simulink model "AME556_Project_Task5"  (R2024b)
settings: Solver=daessc  StartTime=0.0  StopTime=5  FixedStep=0.0005  MaxStep=1e-3  RelTol=1e-2
InitFcn:
  | global params;
  | 
  | % Mass and geometry
  | params.m = 0.25;
  | params.l = 0.22;
  | params.mb = 8;
  | params.a = 0.25;
  | params.b = 0.15;
  | params.g = [0; 9.81; 0];
  | 
  | % Moment of inerita
  | Il_zz = params.m * params.l^2 / 12;
  | Ib_xx = params.mb * params.a^2 / 12;
  | Ib_yy = params.mb * params.b^2 / 12;
  | Ib_zz = params.mb * (params.a^2 + params.b^2) / 12;
  | params.Ib = diag([Ib_xx Ib_yy Ib_zz]);
  | 
  | % Spatial contact force parameters
  | Kp_g = 1e5;
  | Kd_g = 1e3;
  | 
  | % Ground contact positions
  | params.P1 = [0.0197; 0.0022; 0];
  | params.P2 = [0.1838; 0.0041; 0];
  | 
  | % State variables
  | q0 = [0.1; 0.45; 0; -pi/3; pi/2; -pi/6; pi/2]; % Initial states (before landing)
  | params.p_d = [0; 0.5; 0]; % Desired positions (after standing): [x_d; y_d; z_d];
  | params.theta_d = 0; % Desired angle
values from neighbouring files (symbols this model uses):
  dt = 0.04    [AME556_Project_Task5_Setup.m]
  l = 0.5    [AME556_Project_Task5_Setup.m]
  N = 10    [AME556_Project_Task5_Setup.m]
undefined symbols (not defined in the file or in its folder): P1_world0, P2_world0, X, Y, Z
libraries: sm_lib x33, nesl_utility x27
(part 2 of 2)

== matlab function AME556_Project_Task5/MATLAB Function ==
  data: tau_unsaturated input; tau_saturated output; saturateSwitch input
function tau_saturated = tau_saturation(tau_unsaturated, saturateSwitch)
    if saturateSwitch == 1
        tau_limits = [30, 60, 30, 60];
    
        tau_saturated = tau_unsaturated;
    
        for i = 1:length(tau_unsaturated)
            if tau_unsaturated(i) > tau_limits(i)
                tau_saturated(i) = tau_limits(i);
                warning('Tau %d (%.2f) is saturated to %d', i, tau_unsaturated(i), tau_limits(i));
            elseif tau_unsaturated(i) < -tau_limits(i)
                tau_saturated(i) = -tau_limits(i);
                warning('Tau %d (%.2f) is saturated to -%d', i, tau_unsaturated(i), tau_limits(i));
            end
        end
    else
        tau_saturated = tau_unsaturated;
    end
end

== matlab function AME556_Project_Task5/Controller/Condensed MPC Controller ==
  data: p input; theta input; dp input; dtheta input; qs input; tau output; P1 input; P2 input; dP1 input; dP2 input; N input; dt input; t input
%% Function: Low Level Control

function tau = lowLevelControl(p, theta, dp, dtheta, qs, P1, P2, dP1, dP2, N, dt, t)

% 步态的行为应该有：walk run stairs jump_onto_obstacle jump_onto_floor jump_over_pit

if p(1) < 1.8 
    % walk (0,1.8)
    gaitType = "walk";
elseif p(1) < 2.8
    % jump_onto_obstacle (1.8,2.8)
    gaitType = "jump";
elseif p(1) < 4.8
    % jump_onto_floor (2.8,3.8)
elseif p(1) < 5.2
    % jump_over_pit (3.8,4.4)
else
    % walk (4.4,~)
end

con = gaitSchedule(N, dt, t, gaitType);
F = condensed_mpc_controller(p, theta, dp, dtheta, P1, P2, N, dt, t, con, gaitType);
J = jacobianFcn(theta, qs);

tau = zeros(4, 1);
if con(1, 1) && con(2, 1)
    tau = -J' * F;
elseif con(1, 1) && ~con(2, 1)
    F_swing = swingLegControl(p, dp, P2, dP2, N, dt, t, gaitType);
    F_new = [F(1: 2); -F_swing];
    tau = -J' * F_new;
elseif con(2, 1) && ~con(1, 1)
    F_swing = swingLegControl(p, dp, P1, dP1, N, dt, t, gaitType);
    F_new = [-F_swing; F(3: 4)];
    tau = -J' * F_new;    
else
    % 为了飞的修改：俩腿都swing
    F_swing1 = swingLegControl(p, dp, P1, dP1, N, dt, t, gaitType);
    F_swing2 = swingLegControl(p, dp, P2, dP2, N, dt, t, gaitType);
    F_new = [-F_swing1; -F_swing2];
    tau = -J' * F_new;
    % 飞行修改结束
end

end

%% Function: Condensed MPC Controller

function F = condensed_mpc_controller(p, theta, dp, dtheta, P1, P2, N, dt, t, con, gaitType)

    % 为了飞的修改：~any(con(:, 1)) 任何一条腿都不为1（也就是都是0）的话，直接F=0
    if ~any(con(:, 1))
        F = zeros(4, 1); 
        return;
    end
    % 为了飞的修改结束

% Parameters
mt = 8;
a = 0.25;
b = 0.15;
g = [0; 9.81; 0];
Ib_zz = mt * (a^2 + b^2) / 12;

numStates = 7;
numCtrls = 4;
Q = diag([200 200 800 30 10 10 0]);
R = 0.0001*eye(numCtrls);

% q = [x; y; z; R1; dx; dy; dz; wbx; wby; wbz];
% X = [x; y; theta; dx; dy; dtheta; g];
X = zeros(numStates, 1);
X(1: 2) = p;
X(3) = theta;
X(4: 5) = dp;
X(6) = dtheta;
X(7) = g(2);

% Desired states
if gaitType == "walk"
    if t < 1
        X_d = [p_d(1); 0.45; 0; t; 0; 0; g(2)]; % Lower ground walking (acceleration)
    else
        X_d = [p_d(1); 0.45; 0; 1; 0; 0; g(2)]; % Lower ground walking (constant speed)
    end
elseif gaitType == "jump"
    X_d = [p_d(1); 0.4 + 0.45; 0; 1; 0.5; 0; g(2)]; % Going upstairs
end

% Reference Trajectory
X_ref = getReferenceTrajectory(dt, N, p, theta, dp, dtheta, X_d);
y = reshape(X_ref, [numStates*N 1]);

r1 = P1 - p;
r2 = P2 - p;

% Linearized system (A, B)
A = [zeros(3)   eye(3)    zeros(3,1);
     zeros(3, numStates-1) [0; -1; 0];
     zeros(1, numStates)];

B = [zeros(3, numCtrls);
     eye(2)/mt eye(2)/mt;
     -r1(2)/Ib_zz r1(1)/Ib_zz -r2(2)/Ib_zz r2(1)/Ib_zz;
     zeros(1, numCtrls)];

% Discrete-time system matrices (Ak, Bk)
Ak = A * dt + eye(size(A, 1));
Bk = B * dt;

% Aqp
Aqp = [];
for i = 1: N
    Aqp = [Aqp; mpower(Ak, i)];
end

% bqp
Bqp = repmat(zeros(size(Bk)), N, N);
for i = 0: N-1
    element = mpower(Ak, i) * Bk;
    Bqp = Bqp + kron(diag(ones(1, N - i), -i), element);
end

% Condensation
L = kron(eye(N), Q);
K = kron(eye(N), R);

% Optimization weights (H, f)
H = 2*(Bqp'*L*Bqp + K);
f = 2*Bqp'*L*(Aqp*X - y);

% Inequality constraints (A_ineq, b_ineq)
Aineq_mu = kron(eye(2), [1 -0.7; -1 -0.7]);
Aineq_mu_N = kron(eye(N), Aineq_mu);
Aineq_F = kron(eye(2), [0 1; 0 -1]);
Aineq_F_N = kron(eye(N), Aineq_F);
Aineq = [Aineq_mu_N; Aineq_F_N];

bineq_mu = repmat([0; 0; 0; 0], N, 1);
bineq_f = [];
for i = 1: N
    bineq_f = [bineq_f; [250; -10]*con(1, i); [250; -10]*con(2, i)];
end
bineq = [bineq_mu; bineq_f];

% Initial guess
u0 = zeros(length(f), 1);

% Quadratic programming
options = optimoptions('quadprog', 'Algorithm', 'active-set', 'Display', 'off');
u_mpc = quadprog(H, f, Aineq, bineq, [], [], [], [], u0, options);

% Force inputs
F = u_mpc(1: numCtrls);

end

%% Function: Get Reference Geometry

function X_ref = getReferenceTrajectory(dt, N, p, theta, dp, dtheta, X_d)

X = [p; theta; dp; dtheta; 9.81];
X_ref = repmat(X, 1, N);

for i = 1: 3
    for k = 2: N
        if X_d(i + 3) ~= 0
            X_ref(i, k) = X(i) + X_d(i+3)*((k-1)*dt);
        else
            X_ref(i, k) = X_d(i);
        end
    end
end

end

%% Function: Swing Leg Control

function F_swing = swingLegControl(p, dp, P_swing, dP_swing, P_support, N, dt, t)

Kp = diag([200 300]);
Kd = eye(2)*5;

del_t = N*dt/2; % Time duration of swing phase
ts = rem(t, N*dt/2);

if gaitType == "walk"
    swingHeight = 0.1;
    Px_d = p(1) + (1/2)*del_t*dp(1);
    Py_d = swingHeight * sin(pi*ts/del_t); % Flat ground walking
    disp('walk')

elseif gaitType == "jump"
    swingHeight = 0.4;
    Px_d = p(1) + (1/2)*del_t*dp(1);
    Py_d = P_support(2) + (1/2)*del_t*dp(2) + 2*(sin(pi*ts/del_t))^(1/3)*swingHeight; % Going upstairs
    disp('climb')
    
end

F_swing = Kp*([Px_d; Py_d] - P_swing) + Kd*(0 - dP_swing);

end

%% Function: Jacobian Function
% Convert contact forces to joint torques

function J = jacobianFcn(theta, qs)

l = 0.22;

q1 = qs(1); q2 = qs(2); q3 = qs(3); q4 = qs(4);

J = [l*cos(q1 + q2 + theta) + l*cos(q1 + theta), l*cos(q1 + q2 + theta),                                          0,                      0;
     l*sin(q1 + q2 + theta) + l*sin(q1 + theta), l*sin(q1 + q2 + theta),                                          0,                      0;
                                              0,                      0, l*cos(q3 + q4 + theta) + l*cos(q3 + theta), l*cos(q3 + q4 + theta);
                                              0,                      0, l*sin(q3 + q4 + theta) + l*sin(q3 + theta), l*sin(q3 + q4 + theta)];

end

%% Function: Gait Schedule
% Generate gait schedule based on walking phase

function sigma = gaitSchedule(N, dt, t, gaitType)

    if gaitType == "walk"
        phase = floor(t/dt);
        k = rem(phase, N);
        
        sigma_l0 = [ones(1, N/2) zeros(1, N/2)];
        sigma_r0 = [zeros(1, N/2) ones(1, N/2)];
        
        if k ~= 0
            sigma_l = [sigma_l0(k+1: N) sigma_l0(1: k)];
            sigma_r = [sigma_r0(k+1: N) sigma_r0(1: k)];
        else
            sigma_l = sigma_l0;
            sigma_r = sigma_r0;
        end
        
        sigma = [sigma_l; sigma_r];

    elseif gaitType == "jump"
        phase = floor(t/dt);
        k = rem(phase, N);
        
        sigma_l0 = [1 1 1 1 1 0 0 0 0 0];
        sigma_r0 = [1 1 1 1 1 0 0 0 0 0];
        
        if k ~= 0
            sigma_l = [sigma_l0(k+1: N) sigma_l0(1: k)];
            sigma_r = [sigma_r0(k+1: N) sigma_r0(1: k)];
        else
            sigma_l = sigma_l0;
            sigma_r = sigma_r0;
        end
        
        sigma = [sigma_l; sigma_r];       
    
    end
end

== matlab function AME556_Project_Task5/MATLAB Function1 ==
  data: dq input
function physicalConstrains(dq) 
    % 定义每个关节的速度限制（单位：rad/s）
    jointVelocityLimits = [30, 15, 30, 15];
    
    % 将 dq 从 deg/s 转换为 rad/s
    dq_rad = deg2rad(dq); % 角度 -> 弧度转换

    % 遍历所有关节速度，检测是否超限
    for i = 1:length(dq_rad)
        if abs(dq_rad(i)) > jointVelocityLimits(i)
            warning('Joint %d velocity (%.2f rad/s) exceeds the limit! Limit: %.2f rad/s', ...
                    i, dq_rad(i), jointVelocityLimits(i));
        end
    end
end
